simulink model "new_parameter_estimator"  (R2023a)
settings: Solver=VariableStepAuto  StartTime=0.0  StopTime=T_e  RelTol=1e-3
values from neighbouring files (symbols this model uses):
  C1_253 = zeros(1,11)+1000    [for_the_new_parameter_estimator.m]
  C1_263 = zeros(1,11)+1000    [for_the_new_parameter_estimator.m]
  C1_273 = zeros(1,11)+1000    [for_the_new_parameter_estimator.m]
  C1_283 = zeros(1,11)+1000    [for_the_new_parameter_estimator.m]
  C1_298 = zeros(1,11)+1000    [for_the_new_parameter_estimator.m]
  OCV_253 = zeros(1,11)+4    [for_the_new_parameter_estimator.m]
  OCV_263 = zeros(1,11)+4    [for_the_new_parameter_estimator.m]
  OCV_273 = zeros(1,11)+4    [for_the_new_parameter_estimator.m]
  OCV_283 = zeros(1,11)+4    [for_the_new_parameter_estimator.m]
  OCV_298 = zeros(1,11)+4    [for_the_new_parameter_estimator.m]
  R0_253 = zeros(1,11)    [for_the_new_parameter_estimator.m]
  R0_263 = zeros(1,11)    [for_the_new_parameter_estimator.m]
  R0_273 = zeros(1,11)    [for_the_new_parameter_estimator.m]
  R0_283 = zeros(1,11)    [for_the_new_parameter_estimator.m]
  R0_298 = zeros(1,11)    [for_the_new_parameter_estimator.m]
  R1_253 = zeros(1,11)    [for_the_new_parameter_estimator.m]
  R1_263 = zeros(1,11)    [for_the_new_parameter_estimator.m]
  R1_273 = zeros(1,11)    [for_the_new_parameter_estimator.m]
  R1_283 = zeros(1,11)    [for_the_new_parameter_estimator.m]
  R1_298 = zeros(1,11)    [for_the_new_parameter_estimator.m]
libraries: nesl_utility x8, fl_lib x7, ee_lib x1, spspowerguiLib x1
settings Model: Creator=Lenovo  LastModifiedBy=Lenovo
settings DataIOCC: OutputOption=AdditionalOutputTimes  OutputTimes=SDO_OutputTimes

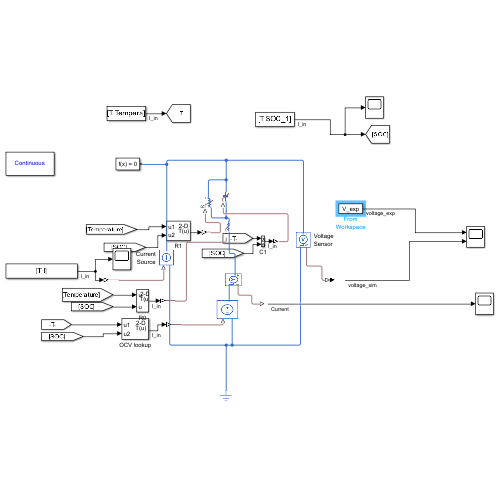
[thumbnail: Simulink's stored preview of the top-level diagram]
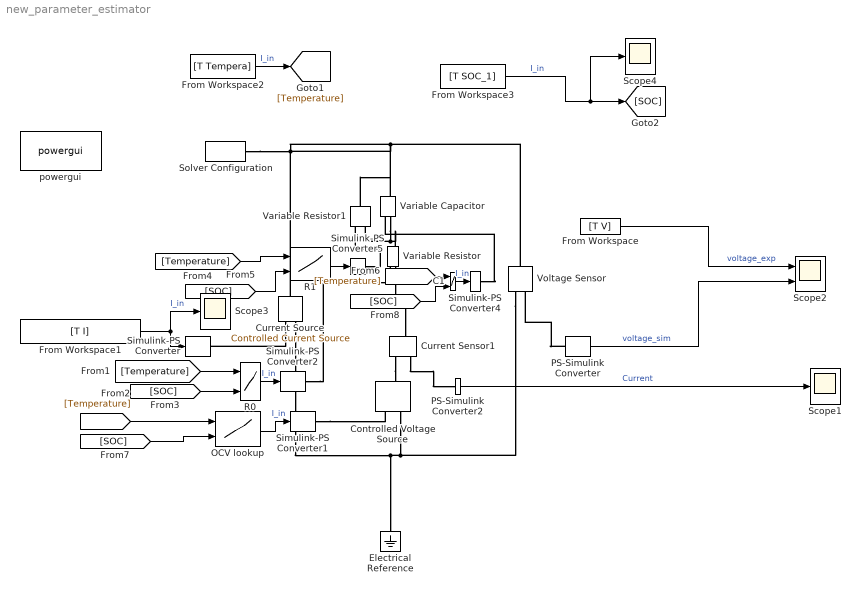
== system new_parameter_estimator ==
  C1 : Lookup_n-D  BreakpointsForDimension1=[253;263;273;283;298]  BreakpointsForDimension2=[0;0.1;0.2;0.3;0.4;0.5;0.6;0.7;0.8;0.9;1]  Table=[C1_253;C1_263;C1_273;C1_283;C1_298]  InternalRulePriority=Speed  RndMeth=Simplest
      settings: InputPortMap=u0,u1
  Controlled Voltage Source : fl_lib/Electrical/Electrical Sources/Controlled Voltage Source
  Current Source : fl_lib/Electrical/Electrical Sources/Controlled Current Source
  Current Sensor1 : fl_lib/Electrical/Electrical Sensors/Current Sensor
  Electrical Reference : fl_lib/Electrical/Electrical Elements/Electrical Reference
  From Workspace : FromWorkspace  VariableName=[T V]
      mask Display: disp('V_exp')
  From Workspace1 : FromWorkspace  VariableName=[T I]
  From Workspace2 : FromWorkspace  VariableName=[T Tempera]
  From Workspace3 : FromWorkspace  VariableName=[T SOC_1]
  OCV lookup : Lookup_n-D  BreakpointsForDimension1=[253;263;273;283;298]  BreakpointsForDimension2=[0;0.1;0.2;0.3;0.4;0.5;0.6;0.7;0.8;0.9;1]  Table=[OCV_253;OCV_263;OCV_273;OCV_283;OCV_298]  InternalRulePriority=Speed  RndMeth=Simplest
      settings: InputPortMap=u0,u1
  PS-Simulink Converter : nesl_utility/PS-Simulink Converter  PhysicalDomain=network_engine_domain  SubClassName=ps_output  LeftPortType=input  RightPortType=output  PseudoPeriodic=off  Frequencies=[]  VectorFormat=1-D array  Unit=V  AffineConversion=off
  PS-Simulink Converter2 : nesl_utility/PS-Simulink Converter  PhysicalDomain=network_engine_domain  SubClassName=ps_output  LeftPortType=input  RightPortType=output  PseudoPeriodic=off  Frequencies=[]  VectorFormat=1-D array  Unit=A  AffineConversion=off
  R0 : Lookup_n-D  BreakpointsForDimension1=[253;263;273;283;298]  BreakpointsForDimension2=[0;0.1;0.2;0.3;0.4;0.5;0.6;0.7;0.8;0.9;1]  Table=[R0_253;R0_263;R0_273;R0_283;R0_298]  InternalRulePriority=Speed  RndMeth=Simplest
      settings: InputPortMap=u0,u1
  R1 : Lookup_n-D  BreakpointsForDimension1=[253;263;273;283;298]  BreakpointsForDimension2=[0;0.1;0.2;0.3;0.4;0.5;0.6;0.7;0.8;0.9;1]  Table=[R1_253;R1_263;R1_273;R1_283;R1_298]  InternalRulePriority=Speed  RndMeth=Simplest
      settings: InputPortMap=u0,u1
  Scope1 : Scope
  Scope2 : Scope  NumInputPorts=2
  Scope3 : Scope
  Scope4 : Scope
  Simulink-PS Converter : nesl_utility/Simulink-PS Converter  PhysicalDomain=network_engine_domain  SubClassName=ps_input  LeftPortType=input  RightPortType=output  PseudoPeriodic=off  Frequencies=[]  NoiseDistribution=none  NoiseParameters=[]  Unit=A  AffineConversion=off  FilteringAndDerivatives=zero  SimscapeFilterOrder=1  InputFilterTimeConstant=.001  UdotUserProvided=0
  Simulink-PS Converter1 : nesl_utility/Simulink-PS Converter  PhysicalDomain=network_engine_domain  SubClassName=ps_input  LeftPortType=input  RightPortType=output  PseudoPeriodic=off  Frequencies=[]  NoiseDistribution=none  NoiseParameters=[]  Unit=V  AffineConversion=off  FilteringAndDerivatives=zero  SimscapeFilterOrder=1  InputFilterTimeConstant=.001  UdotUserProvided=0
  Simulink-PS Converter2 : nesl_utility/Simulink-PS Converter  PhysicalDomain=network_engine_domain  SubClassName=ps_input  LeftPortType=input  RightPortType=output  PseudoPeriodic=off  Frequencies=[]  NoiseDistribution=none  NoiseParameters=[]  Unit=Ohm  AffineConversion=off  FilteringAndDerivatives=zero  SimscapeFilterOrder=1  InputFilterTimeConstant=.001  UdotUserProvided=0
  Simulink-PS Converter4 : nesl_utility/Simulink-PS Converter  PhysicalDomain=network_engine_domain  SubClassName=ps_input  LeftPortType=input  RightPortType=output  PseudoPeriodic=off  Frequencies=[]  NoiseDistribution=none  NoiseParameters=[]  Unit=F  AffineConversion=off  FilteringAndDerivatives=zero  SimscapeFilterOrder=1  InputFilterTimeConstant=.001  UdotUserProvided=0
  Simulink-PS Converter5 : nesl_utility/Simulink-PS Converter  PhysicalDomain=network_engine_domain  SubClassName=ps_input  LeftPortType=input  RightPortType=output  PseudoPeriodic=off  Frequencies=[]  NoiseDistribution=none  NoiseParameters=[]  Unit=Ohm  AffineConversion=on  FilteringAndDerivatives=provide  SimscapeFilterOrder=1  InputFilterTimeConstant=0.001  UdotUserProvided=0
  Solver Configuration : nesl_utility/Solver Configuration  PhysicalDomain=network_engine_domain  SubClassName=solver  LeftPortType=input  RightPortType=generic  Tones=[]  Harmonics=[]  SimulateNoise=off  Profile=off  UseLocalSampling=off  EnableSwitchedLinearOptims=on  FrequencyDomain=off  UseCCode=off  RelTol=0.001  AbsTol=1e-06  MinStep=1e-09  ToWorkspace=off  RevertToSquareIcSolve=off  NumHomotopyIterations=100  PhasorMode=off  PhasorModeNumHarmonics=1  ConsistencySolver=NEWTON_FTOL  IndexReductionMethod=DerivativeReplacement  DoDC=off  ResidualTolerance=1e-9  ConsistencyTolSource=GLOBAL  ConsistencyAbsTol=0.001  ConsistencyRelTol=0.001  ConsistencyTolFactor=0.001  UseLocalSolver=off  LocalSolverChoice=NE_BACKWARD_EULER_ADVANCER  ResolveIndetEquations=on  FunctionEvalNumThread=1  LocalSolverSampleTime=10  DoFixedCost=off  MaxNonlinIter=12  MaxModeIter=2  ComputeImpulses=off  ImpulseIterations=2  LinearAlgebra=Sparse  LinearAlgebraNumThread=0  EquationFormulation=NE_TIME_EF  DelaysMemoryBudget=1024  AutomaticFiltering=on  FilteringTimeConstant=0.001  PartitionStorageMethod=AS_NEEDED  PartitionMemoryBudget=1024  PartitionMethod=FAST
  Variable Capacitor : ee_lib/Passive/Variable Capacitor  prm=2  Cmin=1e-9 F  r=1e-6 Ohm  v0=0 V  q0=0 C
      settings: InternalSimscapePortConfiguration="{\"Bottom\":[],\"Left\":[{\"id\":\"C\",\"label\":\"C\",\"type\":\"input\"},{\"id\":\"p\",\"label\":\"+\",\"type\":\"foundation.electrical.electrical\"}],\"Right\":[{\"id\":\"n\",\"label\":\"-\",\"type\":\"foundation.electrical.electrical\"}],\"Top\":[]}"
  Variable Resistor : fl_lib/Electrical/Electrical Elements/Variable Resistor  Rmin=0 Ohm  i_specify=off  i_priority=None  i=0 A  i_nominal_specify=off  i_nominal_unit=A  i_nominal_value=1  v_specify=off  v_priority=None  v=0 V  v_nominal_specify=off  v_nominal_unit=V  v_nominal_value=1
  Variable Resistor1 : fl_lib/Electrical/Electrical Elements/Variable Resistor  Rmin=0 Ohm  i_specify=off  i_priority=None  i=0 A  i_nominal_specify=off  i_nominal_unit=A  i_nominal_value=1  v_specify=off  v_priority=None  v=0 V  v_nominal_specify=off  v_nominal_unit=V  v_nominal_value=1
  Voltage Sensor : fl_lib/Electrical/Electrical Sensors/Voltage Sensor
  powergui : spspowerguiLib/powergui  Priority=1  SimulationMode=Continuous  SampleTime=50e-6  frequency=60  Iterations=50  frequencyindice=60  Pbase=100e6  ErrMax=1e-4  UnitsV=kV  UnitsW=MW  buscounter=0  FunctionMessages=off  echomessages=off  EnableUseOfTLC=off  CurrentSourceSwitches=off  DisableSnubberDevices=off  DisableRonSwitches=off  DisableVfSwitches=off  DisplayEquations=off  AutomaticDiscreteSolvers=off  SolverType=Tustin/Backward Euler (TBE)  Interpol=off  ExternalGateDelay=off  methode=off  Ts=100  x0status=blocks  SPID=on  SwTol=0  HookPort=off  NonlinearTolerance=1e-4  nMaxIteration=100  ContinueOnMaxIteration=off  RestoreLinks=warning  ResistiveCurrentMeasurement=off  Frange=[0:2:500]  Ylog=off  Xlog=on  ShowGrid=off  save=off  variable=ZData  structure=0  ZoomFFT=off  StartTime=0.0  cycles=1  DisplayStyle=1  fundamental=60  FreqAxis=off  MaxFrequency=1000  frequencyindicesteady=1  RmsSteady=1  display=off
  wires:
  R0/1 -> Simulink-PS Converter2/1  "I_in"
  C1/1 -> Simulink-PS Converter4/1  "I_in"
  R1/1 -> Simulink-PS Converter5/1
  OCV lookup/1 -> Simulink-PS Converter1/1  "I_in"
  PS-Simulink Converter/1 -> Scope2/2  "voltage_sim"
  From Workspace/1 -> Scope2/1  "voltage_exp"
  [Temperature] -> OCV lookup/1
  [SOC] -> OCV lookup/2
  [Temperature] -> R0/1
  [SOC] -> R0/2
  [Temperature] -> R1/1
  [SOC] -> R1/2
  [Temperature] -> C1/1
  [SOC] -> C1/2
  From Workspace2/1 -> [Temperature]  "I_in"
  From Workspace1/1 -> Simulink-PS Converter/1, Scope3/1  "I_in"
  PS-Simulink Converter2/1 -> Scope1/1  "Current"
  From Workspace3/1 -> Scope4/1, [SOC]  "I_in"
  connections:
  Solver Configuration/RConn1 -- Current Source/LConn1 -- Voltage Sensor/LConn1 -- Variable Resistor1/RConn1 -- Variable Capacitor/RConn1
  Variable Capacitor/LConn2 -- Variable Resistor/RConn1 -- Variable Resistor1/LConn2
  Voltage Sensor/RConn2 -- Current Source/RConn2 -- Electrical Reference/LConn1 -- Controlled Voltage Source/RConn2
  PS-Simulink Converter/LConn1 -- Voltage Sensor/RConn1
  Simulink-PS Converter1/RConn1 -- Controlled Voltage Source/RConn1
  Simulink-PS Converter2/RConn1 -- Variable Resistor/LConn1
  Simulink-PS Converter4/RConn1 -- Variable Capacitor/LConn1
  Current Source/RConn1 -- Simulink-PS Converter/RConn1
  Simulink-PS Converter5/RConn1 -- Variable Resistor1/LConn1
  Current Sensor1/RConn2 -- Controlled Voltage Source/LConn1
  Variable Resistor/LConn2 -- Current Sensor1/LConn1
  Current Sensor1/RConn1 -- PS-Simulink Converter2/LConn1
